simulink model "Fire_Detection_WebCam"  (R2023b)
settings: Solver=FixedStepAuto  StartTime=0.0  StopTime=60  RelTol=1e-3
undefined symbols (not defined in the file or in its folder): gray, none, videoinput
libraries: imaqlib x1
settings Model: Creator=Amir  LastModifiedBy=vahed
settings SolverCC: AlgebraicLoopSolver=TrustRegion
settings DataIOCC: ReturnWorkspaceOutputs=off
settings DebuggingCC: UnconnectedInputMsg=warning  UnconnectedOutputMsg=warning  UnconnectedLineMsg=warning  ArithmeticOperatorsInVariantConditions=warning
settings HardwareCC: ProdBitPerLong=64  ProdHWDeviceType=Intel->x86-64 (Linux 64)
settings ModelReferenceCC: EnableRefExpFcnMdlSchedulingChecks=on
settings SFSimCC: CustomCodeUndefinedFunction=UseInterfaceOnly
settings RTWCC: Description=Simulink Desktop Real-Time  SystemTargetFile=sldrt.tlc  TemplateMakefile=sldrt.tmf  RTWCompilerOptimization=on  DLArmComputeVersion=19.05
settings CodeAppCC: MaxIdLength=95
settings SimulinkDesktopRealTimeCC: TargetLibSuffix=_sldrt.a  TargetPreCompLibLocation=C:\MATLAB\R2023b\toolbox\sldrt\lib\win64  CodeReplacementLibrary=GNU C99 extensions

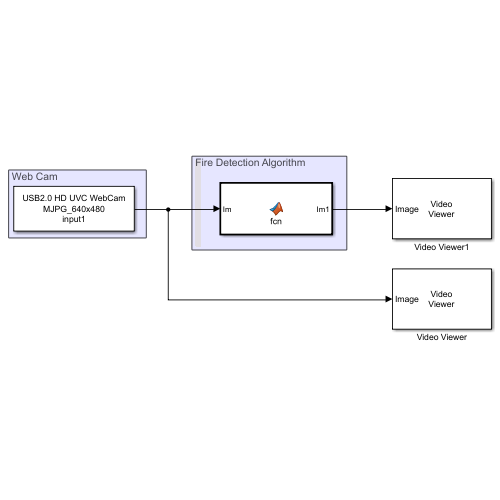
[thumbnail: Simulink's stored preview of the top-level diagram]
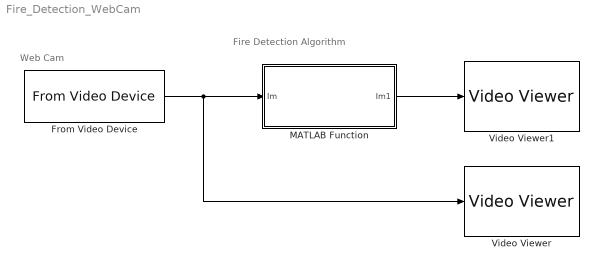
== system Fire_Detection_WebCam ==
  note: Fire Detection Algorithm
  note: Web Cam
  From Video Device : imaqlib/From Video Device  DeviceMenu=(none)  Device=winvideo 1 (USB2.0 HD UVC WebCam)  ObjConstructor=videoinput('winvideo', 1)  VideoFormatMenu=(none)  VideoFormat=MJPG_640x480  VideoSource=input1  ROIPosition=[0 0 480 640]  EnableHWTrigger=off  TriggerConfiguration=none/none  SampleTime=0.01  OutputPortsMode=One multidimensional signal  DataType=double  CanDoHWTrigger=no  ReturnedColorSpace=rgb  BlockHandle=17.0001  ROIWidth=640  ROIHeight=480  ROIColumn=0  ROIRow=0  EngXMLPath=C:\MATLAB\R2023b\toolbox\imaq\imaq\private  DevXMLPath=C:\ProgramData\MATLAB\SupportPackages\R2023b\toolbox\imaq\supportpackages\genericvideo\adaptor\win64  EngLibPath=C:\MATLAB\R2023b\toolbox\imaq\imaqblks\imaqmex\win64  ColorSpace=rgb  BayerSensorAlignment=grbg  ImaqMode=off
  MATLAB Function : MATLAB Function  TreatAsAtomicUnit=on
  Video Viewer : VideoViewer  colormapValue=gray(256)  FigPos=[35.4 742.8 675.2 508.8]
  Video Viewer1 : VideoViewer  colormapValue=gray(256)  FigPos=[715.4 743.6 742.4 504.8]
  wires:
  MATLAB Function/1(Im1) -> Video Viewer1/1
  From Video Device/1 -> Video Viewer/1, MATLAB Function/1(Im)

== matlab function Fire_Detection_WebCam/MATLAB Function ==
  data: Im input; Im1 output
function Im1 = fcn(Im)
Im=Im.*255;
[m,n,~]=size(Im);
mask=zeros(m,n);
Im_LAB = rgb2lab(Im);
Lm=mean(mean(Im_LAB(:,:,1)));
Am=mean(mean(Im_LAB(:,:,2)));
Bm=mean(mean(Im_LAB(:,:,3)));
R_T=230;%[115 135]
for i=1:m
    for j=1:n
        if Im(i,j,1)>=R_T
            if Im(i,j,1)>=Im(i,j,2) && Im(i,j,2)>=Im(i,j,3)
                if Im(i,j,2)/(Im(i,j,1)+255)>=0.25 && Im(i,j,2)/(Im(i,j,1)+255)<=0.65
                    if Im(i,j,3)/(Im(i,j,1)+255)>=0.05 && Im(i,j,3)/(Im(i,j,1)+255)<=0.45
                        if Im(i,j,3)/(Im(i,j,2)+255)>=0.2 && Im(i,j,3)/(Im(i,j,2)+255)<=0.6
                            if Im_LAB(i,j,1)>=Lm && Im_LAB(i,j,2)>=Am && Im_LAB(i,j,3)>=Bm %&& Im_LAB(i,j,3)>=Im_LAB(i,j,2)
                                mask(i,j)=1;
                            end
                        end
                    end
                end
            end
        end
    end
end
Im1= bsxfun(@times, Im, cast(mask, 'like', Im))./255;
% Im1=mask;
